simulink model "Thermoelectric_Regen_Damper"  (R2020a)
settings: Solver=VariableStepAuto  StartTime=0.0  StopTime=10.0  RelTol=1e-3
libraries: powerlib x13
settings Model: Creator=Aditya Sharma  LastModifiedBy=Aditya Sharma

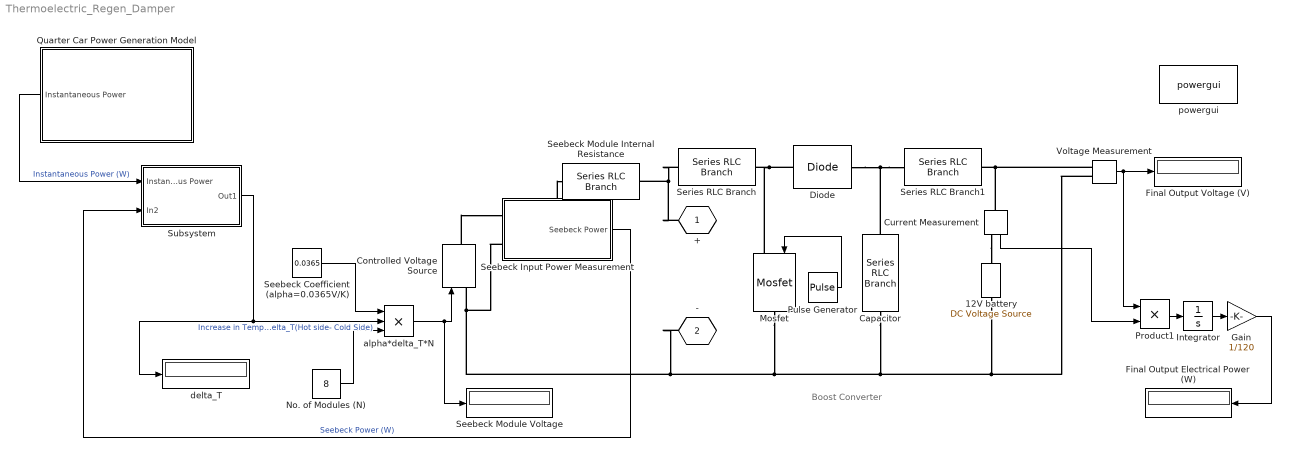
== system Thermoelectric_Regen_Damper ==
  note: Boost Converter
  12V battery : powerlib/Electrical Sources/DC Voltage Source  Amplitude=12  Measurements=None
  Capacitor : powerlib/Elements/Series RLC Branch  LConnTagsString=__new0  RConnTagsString=__new0  BranchType=C  Resistance=1  Inductance=1e-3  SetiL0=off  InitialCurrent=0  Capacitance=7.68*10^-6  Setx0=off  InitialVoltage=0  Measurements=None
  Controlled Voltage Source : powerlib/Electrical Sources/Controlled Voltage Source  Initialize=on  Source_Type=AC  Amplitude=0  Phase=0  Frequency=0  Measurements=None
  Current Measurement : powerlib/Measurements/Current Measurement  PhasorSimulation=off  OutputType=Complex  PSBequivalent=0
  Diode : powerlib/Power Electronics/Diode  Ron=0.001  Lon=0  Vf=0.8  IC=0  UseSnubber=0  Rs=500  Cs=250e-9  Measurements=off
  Final Output Voltage (V) : Display
  Final Output Electrical Power (W) : Display
  Gain : Gain  Gain=1/120
  Integrator : Integrator
  Mosfet : powerlib/Power Electronics/Mosfet  Ron=0.001  Lon=0  Rd=0.01  Vfd=0  IC=0  Rs=1e5  Cs=inf  Measurements=off
  No. of Modules (N) : Constant  Value=8
  Product1 : Product
  Pulse Generator : DiscretePulseGenerator  PulseType=Time based  Period=3.2e-5  PulseWidth=91.6667
  Quarter Car Power Generation Model : Subsystem
  Seebeck Coefficient (alpha=0.0365V/K) : Constant  Value=0.0365
  "Seebeck Input Power Measurement " : Subsystem
      settings: PortSchema="{\"entries\":[{\"content\":{\"sides\":[{\"content\":{\"connectorIds\":[\"LConn1\",\"LConn2\"]},\"type\":\"ConnectorPlacement.EquallySpacedRectSide\",\"uuid\":\"da9ecea4-fa10-45b5-a8cf-d5f181d74830\"},{\"content\":{\"connectorIds\":[\"Out1\"],\"side\":\"RIGHT\"},\"type\":\"ConnectorPlacement.EquallySpacedRectSide\",\"uuid\":\"87535208-3128-4425-91ba-3b63ced5399f\"},{\"content\":{\"connectorIds\":[\"LConn3\"],\"side\":\"TOP\"},\"type\":\"ConnectorPlacement.EquallySpacedRectSide\",\"uuid\":\"5c6a1d2d-c134-4837-8d9e-c0d560ec347a\"}]},\"type\":\"ConnectorPlacement.EquallySpacedConnector\",\"uuid\":\"8daf93c7-3ae1-480e-8d20-21c816cf2981\"}],\"packageUris\":[\"http://schema.mathworks.com/mf0/Connector/19700101\"],\"version\":\"1.0\"}"
  Seebeck Module Internal Resistance : powerlib/Elements/Series RLC Branch  LConnTagsString=__new0  RConnTagsString=__new0  BranchType=R  Resistance=0.7  Inductance=1e-3  SetiL0=off  InitialCurrent=0  Capacitance=1e-6  Setx0=off  InitialVoltage=0  Measurements=None
  Seebeck Module Voltage : Display
  Series RLC Branch : powerlib/Elements/Series RLC Branch  LConnTagsString=__new0  RConnTagsString=__new0  BranchType=L  Resistance=1  Inductance=1e-4  SetiL0=off  InitialCurrent=0  Capacitance=1e-6  Setx0=off  InitialVoltage=0  Measurements=None
  Series RLC Branch1 : powerlib/Elements/Series RLC Branch  LConnTagsString=__new0  RConnTagsString=__new0  BranchType=RL  Resistance=0.02  Inductance=1e-4  SetiL0=off  InitialCurrent=0  Capacitance=1e-6  Setx0=off  InitialVoltage=0  Measurements=None
  Subsystem : Subsystem
  Voltage Measurement : powerlib/Measurements/Voltage Measurement  PhasorSimulation=off  OutputType=Complex  PSBequivalent=0
  alpha*delta_T*N : Product  Inputs=3
  delta_T : Display
  powergui : powerlib/powergui  Priority=1  SimulationMode=Continuous  SampleTime=1e-4  frequency=60  Iterations=50  frequencyindice=0  Pbase=100e6  ErrMax=1e-4  UnitsV=kV  UnitsW=MW  buscounter=0  FunctionMessages=off  echomessages=off  EnableUseOfTLC=off  CurrentSourceSwitches=off  DisableSnubberDevices=off  DisableRonSwitches=off  DisableVfSwitches=off  DisplayEquations=off  AutomaticDiscreteSolvers=off  SolverType=Tustin/Backward Euler (TBE)  Interpol=off  ExternalGateDelay=off  methode=off  Ts=100  x0status=blocks  SPID=on  SwTol=0  HookPort=off  NonlinearTolerance=1e-4  nMaxIteration=100  ContinueOnMaxIteration=off  RestoreLinks=warning  ResistiveCurrentMeasurement=off  Frange=[0:2:500]  Ylog=off  Xlog=on  ShowGrid=off  save=off  variable=ZData  structure=0  ZoomFFT=off  StartTime=0.0  cycles=1  DisplayStyle=1  fundamental=60  FreqAxis=off  MaxFrequency=1000  frequencyindicesteady=1  RmsSteady=1  display=off
  + : PMIOPort  Tag=PMCPort  Side=Right
  - : PMIOPort  Tag=PMCPort  Port=2  Side=Right
  wires:
  Gain/1 -> Final Output Electrical Power (W)/1
  alpha*delta_T*N/1 -> Controlled Voltage Source/1, Seebeck Module Voltage/1
  Product1/1 -> Integrator/1
  Subsystem/1(Out1) -> delta_T/1, alpha*delta_T*N/2  "Increase in Temperature delta_T(Hot side- Cold Side)"
  "Seebeck Input Power Measurement "/1(Seebeck Power) -> Subsystem/2(In2)  "Seebeck Power (W)"
  Integrator/1 -> Gain/1
  Current Measurement/1 -> Product1/2
  Voltage Measurement/1 -> Product1/1, Final Output Voltage (V)/1
  Quarter Car Power Generation Model/1("Instantaneous Power ") -> Subsystem/1(Instantaneous Power)  "Instantaneous Power (W)"
  No. of Modules (N)/1 -> alpha*delta_T*N/3
  Pulse Generator/1 -> Mosfet/1
  Seebeck Coefficient (alpha=0.0365V/K)/1 -> alpha*delta_T*N/1
  connections:
  Controlled Voltage Source/LConn1 -- "Seebeck Input Power Measurement "/LConn2 -- Voltage Measurement/LConn2 -- 12V battery/LConn1 -- Capacitor/LConn1 -- Mosfet/RConn1 -- -/RConn1
  Seebeck Module Internal Resistance/RConn1 -- Series RLC Branch/LConn1 -- +/RConn1
  Series RLC Branch1/RConn1 -- Voltage Measurement/LConn1 -- Current Measurement/LConn1
  Series RLC Branch1/LConn1 -- Diode/RConn1 -- Capacitor/RConn1
  Series RLC Branch/RConn1 -- Mosfet/LConn1 -- Diode/LConn1
  Controlled Voltage Source/RConn1 -- "Seebeck Input Power Measurement "/LConn1
  Current Measurement/RConn1 -- 12V battery/RConn1
  "Seebeck Input Power Measurement "/LConn3 -- Seebeck Module Internal Resistance/LConn1

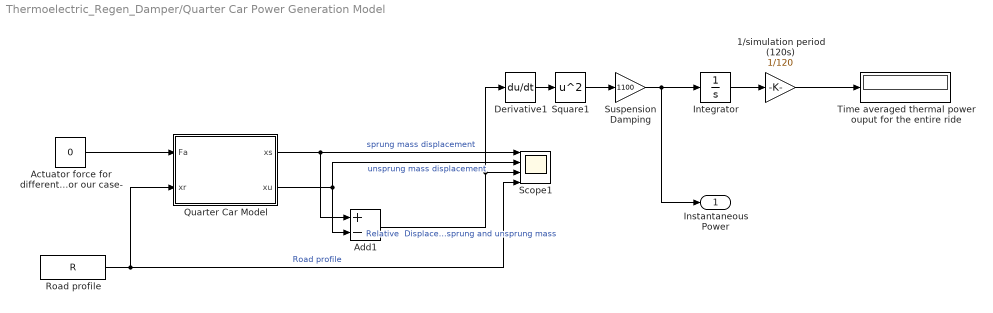
== system Thermoelectric_Regen_Damper/Quarter Car Power Generation Model ==
  1/simulation period (120s) : Gain  Gain=1/120
  "Actuator force for different types of suspension -zero for our case- " : Constant  Value=0
  Add1 : Sum  Inputs=+-
  Derivative1 : Derivative
  Integrator : Integrator
  Quarter Car Model : Subsystem
  Road profile : FromWorkspace  VariableName=R
  Scope1 : Scope  NumInputPorts=4
  Square1 : Math  Operator=square  SaturateOnIntegerOverflow=on
  Suspension Damping : Gain  Gain=1100
  "Time averaged thermal power ouput for the entire ride " : Display
  "Instantaneous Power " : Outport
  wires:
  1/simulation period (120s)/1 -> "Time averaged thermal power ouput for the entire ride "/1
  Square1/1 -> Suspension Damping/1
  "Actuator force for different types of suspension -zero for our case- "/1 -> Quarter Car Model/1(Fa)
  Suspension Damping/1 -> "Instantaneous Power "/1, Integrator/1
  Road profile/1 -> Quarter Car Model/2(xr), Scope1/4  "Road profile"
  Quarter Car Model/1(xs) -> Add1/1, Scope1/1  "sprung mass displacement"
  Integrator/1 -> 1/simulation period (120s)/1
  Derivative1/1 -> Square1/1
  Add1/1 -> Derivative1/1, Scope1/3  "Relative  Displacement b/w sprung and unsprung mass"
  Quarter Car Model/2(xu) -> Scope1/2, Add1/2  "unsprung mass displacement"

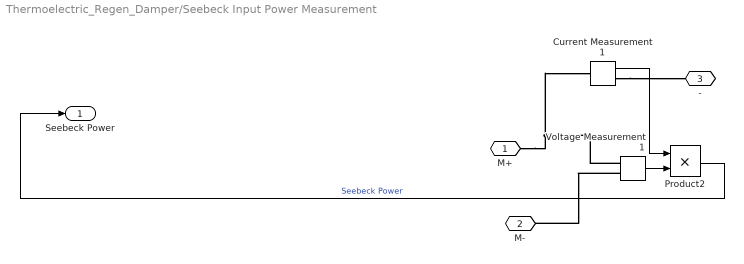
== system Thermoelectric_Regen_Damper/Seebeck Input Power Measurement  ==
  Current Measurement1 : powerlib/Measurements/Current Measurement  PhasorSimulation=off  OutputType=Complex  PSBequivalent=0
  Product2 : Product
  Voltage Measurement1 : powerlib/Measurements/Voltage Measurement  PhasorSimulation=off  OutputType=Complex  PSBequivalent=0
  M+ : PMIOPort  Side=Left
  M- : PMIOPort  Port=2  Side=Left
  - : PMIOPort  Port=3  Side=Left
  Seebeck Power : Outport
  wires:
  Voltage Measurement1/1 -> Product2/2
  Product2/1 -> Seebeck Power/1  "Seebeck Power"
  Current Measurement1/1 -> Product2/1
  connections:
  M+/RConn1 -- Voltage Measurement1/LConn1 -- Current Measurement1/LConn1
  Current Measurement1/RConn1 -- -/RConn1
  Voltage Measurement1/LConn2 -- M-/RConn1

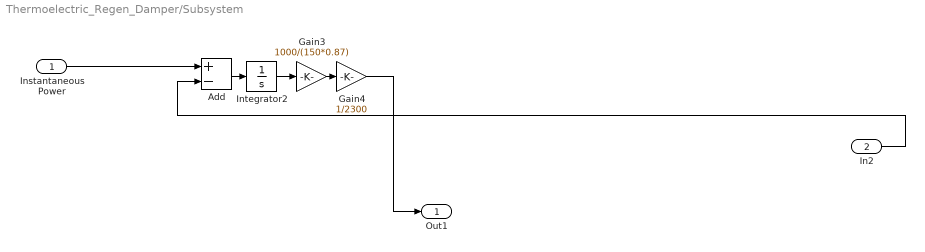
== system Thermoelectric_Regen_Damper/Subsystem ==
  Instantaneous Power : Inport
  In2 : Inport  Port=2
  Add : Sum  Inputs=+-
  Gain3 : Gain  Gain=1000/(150*0.87)
  Gain4 : Gain  Gain=1/2300
  Integrator2 : Integrator
  Out1 : Outport
  wires:
  Gain3/1 -> Gain4/1
  Add/1 -> Integrator2/1
  Integrator2/1 -> Gain3/1
  Instantaneous Power/1 -> Add/1
  In2/1 -> Add/2
  Gain4/1 -> Out1/1

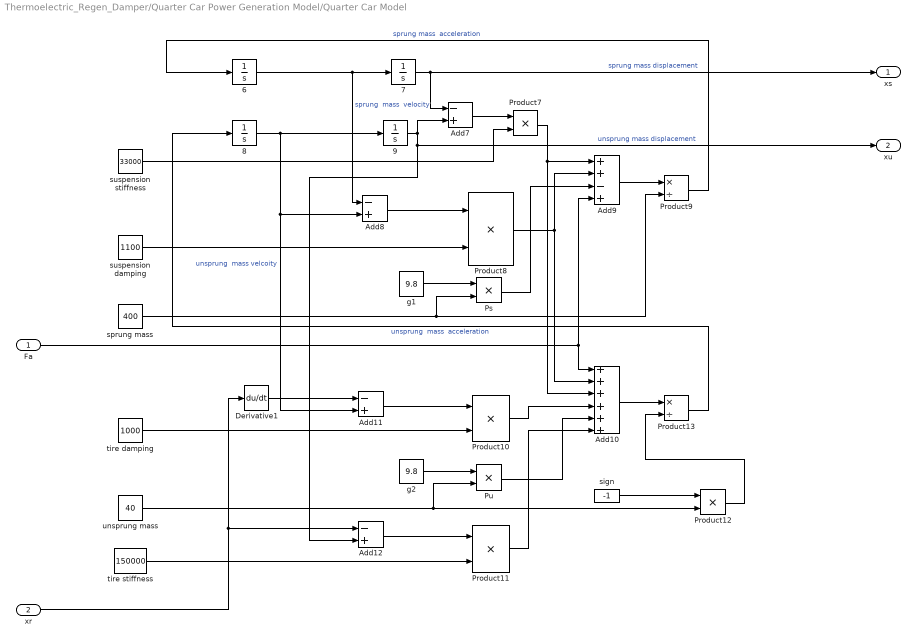
== system Thermoelectric_Regen_Damper/Quarter Car Power Generation Model/Quarter Car Model ==
  Fa : Inport
  xr : Inport  Port=2
  {6..9} (4 alike) : Integrator
  Add10 : Sum  Inputs=++++++
  Add{7..8,11..12} (4 alike) : Sum  Inputs=-+
  Add9 : Sum  Inputs=++-+
  Derivative1 : Derivative
  Product{7..8,10..12} (5 alike) : Product
  Product13 : Product  Inputs=*/
  Product9 : Product  Inputs=*/
  Ps : Product
  Pu : Product
  g1 : Constant  Value=9.8
  g2 : Constant  Value=9.8
  sign : Constant  Value=-1
  sprung mass : Constant  Value=400
  suspension damping : Constant  Value=1100
  suspension stiffness : Constant  Value=33000
  "tire damping " : Constant  Value=1000
  tire stiffness : Constant  Value=150000
  unsprung mass : Constant  Value=40
  xs : Outport
  xu : Outport  Port=2
  wires:
  g1/1 -> Ps/1
  Product12/1 -> Product13/2
  g2/1 -> Pu/1
  Ps/1 -> Add9/3
  Add10/1 -> Product13/1
  sign/1 -> Product12/1
  unsprung mass/1 -> Pu/2, Product12/2
  Product11/1 -> Add10/6
  Add12/1 -> Product11/1
  tire stiffness/1 -> Product11/2
  xr/1 -> Add12/1, Derivative1/1
  Pu/1 -> Add10/5
  Product10/1 -> Add10/4
  Add11/1 -> Product10/1
  "tire damping "/1 -> Product10/2
  Derivative1/1 -> Add11/1
  sprung mass/1 -> Product9/2, Ps/2
  Add9/1 -> Product9/1
  Fa/1 -> Add10/1, Add9/4
  Product8/1 -> Add10/2, Add9/2
  Product7/1 -> Add10/3, Add9/1
  suspension damping/1 -> Product8/2
  Add8/1 -> Product8/1
  suspension stiffness/1 -> Product7/2
  Add7/1 -> Product7/1
  9/1 -> Add12/2, xu/1, Add7/2  "unsprung mass displacement"
  Product13/1 -> 8/1  "unsprung  mass  acceleration"
  8/1 -> 9/1, Add8/2, Add11/2  "unsprung  mass velcoity"
  7/1 -> Add7/1, xs/1  "sprung mass displacement"
  Product9/1 -> 6/1  "sprung mass  acceleration"
  6/1 -> 7/1, Add8/1  "sprung  mass  velocity"
